simulink model "TST_HLSDem_SelectParameter"  (R2016b)
settings: Solver=FixedStepDiscrete  StartTime=0.0  StopTime=simTime  FixedStep=sampleTime  RelTol=1e-3
values from neighbouring files (symbols this model uses):
  testCase = 1    [initTST_HLSDem_SelectParameter_001.m]    (also in initTST_HLSDem_SelectParameter_002.m = 2; initTST_HLSDem_SelectParameter_003.m = 3; initTST_HLSDem_SelectParameter_004.m = 4; initTST_HLSDem_SelectParameter_005.m = 5)
libraries: simulink x146, UnitTest_Lib x140
(part 1 of 4)
settings Model: Creator=caijinkang  LastModifiedBy=caijinkang
settings DebuggingCC: SignalRangeChecking=error

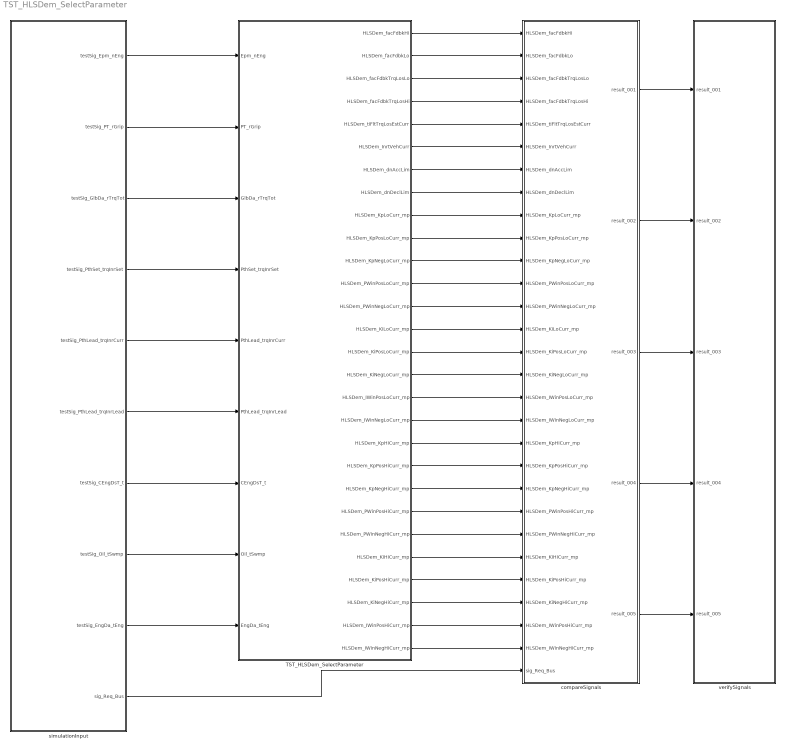
== system TST_HLSDem_SelectParameter ==
  TST_HLSDem_SelectParameter : Subsystem
  compareSignals : Subsystem
  simulationInput : Subsystem
  verifySignals : Subsystem
  wires:
  simulationInput/1(testSig_Epm_nEng) -> TST_HLSDem_SelectParameter/1(Epm_nEng)
  simulationInput/2(testSig_PT_rGrip) -> TST_HLSDem_SelectParameter/2(PT_rGrip)
  simulationInput/3(testSig_GlbDa_rTrqTot) -> TST_HLSDem_SelectParameter/3(GlbDa_rTrqTot)
  simulationInput/4(testSig_PthSet_trqInrSet) -> TST_HLSDem_SelectParameter/4(PthSet_trqInrSet)
  simulationInput/5(testSig_PthLead_trqInrCurr) -> TST_HLSDem_SelectParameter/5(PthLead_trqInrCurr)
  simulationInput/6(testSig_PthLead_trqInrLead) -> TST_HLSDem_SelectParameter/6(PthLead_trqInrLead)
  simulationInput/7(testSig_CEngDsT_t) -> TST_HLSDem_SelectParameter/7(CEngDsT_t)
  simulationInput/8(testSig_Oil_tSwmp) -> TST_HLSDem_SelectParameter/8(Oil_tSwmp)
  simulationInput/9(testSig_EngDa_tEng) -> TST_HLSDem_SelectParameter/9(EngDa_tEng)
  TST_HLSDem_SelectParameter/1(HLSDem_facFdbkHi) -> compareSignals/1(HLSDem_facFdbkHi)
  TST_HLSDem_SelectParameter/2(HLSDem_facFdbkLo) -> compareSignals/2(HLSDem_facFdbkLo)
  TST_HLSDem_SelectParameter/3(HLSDem_facFdbkTrqLosLo) -> compareSignals/3(HLSDem_facFdbkTrqLosLo)
  TST_HLSDem_SelectParameter/4(HLSDem_facFdbkTrqLosHi) -> compareSignals/4(HLSDem_facFdbkTrqLosHi)
  TST_HLSDem_SelectParameter/5(HLSDem_tiFltTrqLosEstCurr) -> compareSignals/5(HLSDem_tiFltTrqLosEstCurr)
  TST_HLSDem_SelectParameter/6(HLSDem_InrtVehCurr) -> compareSignals/6(HLSDem_InrtVehCurr)
  TST_HLSDem_SelectParameter/7(HLSDem_dnAccLim) -> compareSignals/7(HLSDem_dnAccLim)
  TST_HLSDem_SelectParameter/8(HLSDem_dnDeclLim) -> compareSignals/8(HLSDem_dnDeclLim)
  TST_HLSDem_SelectParameter/9(HLSDem_KpLoCurr_mp) -> compareSignals/9(HLSDem_KpLoCurr_mp)
  TST_HLSDem_SelectParameter/10(HLSDem_KpPosLoCurr_mp) -> compareSignals/10(HLSDem_KpPosLoCurr_mp)
  TST_HLSDem_SelectParameter/11(HLSDem_KpNegLoCurr_mp) -> compareSignals/11(HLSDem_KpNegLoCurr_mp)
  TST_HLSDem_SelectParameter/12(HLSDem_PWinPosLoCurr_mp) -> compareSignals/12(HLSDem_PWinPosLoCurr_mp)
  TST_HLSDem_SelectParameter/13(HLSDem_PWinNegLoCurr_mp) -> compareSignals/13(HLSDem_PWinNegLoCurr_mp)
  TST_HLSDem_SelectParameter/14(HLSDem_KiLoCurr_mp) -> compareSignals/14(HLSDem_KiLoCurr_mp)
  TST_HLSDem_SelectParameter/15(HLSDem_KiPosLoCurr_mp) -> compareSignals/15(HLSDem_KiPosLoCurr_mp)
  TST_HLSDem_SelectParameter/16(HLSDem_KiNegLoCurr_mp) -> compareSignals/16(HLSDem_KiNegLoCurr_mp)
  TST_HLSDem_SelectParameter/17(HLSDem_IWinPosLoCurr_mp) -> compareSignals/17(HLSDem_IWinPosLoCurr_mp)
  TST_HLSDem_SelectParameter/18(HLSDem_IWinNegLoCurr_mp) -> compareSignals/18(HLSDem_IWinNegLoCurr_mp)
  TST_HLSDem_SelectParameter/19(HLSDem_KpHiCurr_mp) -> compareSignals/19(HLSDem_KpHiCurr_mp)
  TST_HLSDem_SelectParameter/20(HLSDem_KpPosHiCurr_mp) -> compareSignals/20(HLSDem_KpPosHiCurr_mp)
  TST_HLSDem_SelectParameter/21(HLSDem_KpNegHiCurr_mp) -> compareSignals/21(HLSDem_KpNegHiCurr_mp)
  TST_HLSDem_SelectParameter/22(HLSDem_PWinPosHiCurr_mp) -> compareSignals/22(HLSDem_PWinPosHiCurr_mp)
  TST_HLSDem_SelectParameter/23(HLSDem_PWinNegHiCurr_mp) -> compareSignals/23(HLSDem_PWinNegHiCurr_mp)
  TST_HLSDem_SelectParameter/24(HLSDem_KiHiCurr_mp) -> compareSignals/24(HLSDem_KiHiCurr_mp)
  TST_HLSDem_SelectParameter/25(HLSDem_KiPosHiCurr_mp) -> compareSignals/25(HLSDem_KiPosHiCurr_mp)
  TST_HLSDem_SelectParameter/26(HLSDem_KiNegHiCurr_mp) -> compareSignals/26(HLSDem_KiNegHiCurr_mp)
  TST_HLSDem_SelectParameter/27(HLSDem_IWinPosHiCurr_mp) -> compareSignals/27(HLSDem_IWinPosHiCurr_mp)
  TST_HLSDem_SelectParameter/28(HLSDem_IWinNegHiCurr_mp) -> compareSignals/28(HLSDem_IWinNegHiCurr_mp)
  simulationInput/10(sig_Req_Bus) -> compareSignals/29(sig_Req_Bus)
  compareSignals/1(result_001) -> verifySignals/1(result_001)
  compareSignals/2(result_002) -> verifySignals/2(result_002)
  compareSignals/3(result_003) -> verifySignals/3(result_003)
  compareSignals/4(result_004) -> verifySignals/4(result_004)
  compareSignals/5(result_005) -> verifySignals/5(result_005)

== system TST_HLSDem_SelectParameter/TST_HLSDem_SelectParameter ==
  Epm_nEng : Inport
  PT_rGrip : Inport  Port=2
  GlbDa_rTrqTot : Inport  Port=3
  PthSet_trqInrSet : Inport  Port=4
  PthLead_trqInrCurr : Inport  Port=5
  PthLead_trqInrLead : Inport  Port=6
  CEngDsT_t : Inport  Port=7
  Oil_tSwmp : Inport  Port=8
  EngDa_tEng : Inport  Port=9
  Function_Call : simulink/Ports & Subsystems/Function-Call Generator  sample_time=sampleTime  numberOfIterations=1
  HLSDem_SelectParameter : ModelReference  ModelNameDialog=HLSDem_SelectParameter  SimulationMode=Normal  ModelReferenceVersion=1.85  TriggerPortName=function  TriggerPortTriggerType=function-call  TriggerPortStatesWhenEnabling=held
  HLSDem_facFdbkHi : Outport
  HLSDem_facFdbkLo : Outport  Port=2
  HLSDem_facFdbkTrqLosLo : Outport  Port=3
  HLSDem_facFdbkTrqLosHi : Outport  Port=4
  HLSDem_tiFltTrqLosEstCurr : Outport  Port=5
  HLSDem_InrtVehCurr : Outport  Port=6
  HLSDem_dnAccLim : Outport  Port=7
  HLSDem_dnDeclLim : Outport  Port=8
  HLSDem_KpLoCurr_mp : Outport  Port=9
  HLSDem_KpPosLoCurr_mp : Outport  Port=10
  HLSDem_KpNegLoCurr_mp : Outport  Port=11
  HLSDem_PWinPosLoCurr_mp : Outport  Port=12
  HLSDem_PWinNegLoCurr_mp : Outport  Port=13
  HLSDem_KiLoCurr_mp : Outport  Port=14
  HLSDem_KiPosLoCurr_mp : Outport  Port=15
  HLSDem_KiNegLoCurr_mp : Outport  Port=16
  HLSDem_IWinPosLoCurr_mp : Outport  Port=17
  HLSDem_IWinNegLoCurr_mp : Outport  Port=18
  HLSDem_KpHiCurr_mp : Outport  Port=19
  HLSDem_KpPosHiCurr_mp : Outport  Port=20
  HLSDem_KpNegHiCurr_mp : Outport  Port=21
  HLSDem_PWinPosHiCurr_mp : Outport  Port=22
  HLSDem_PWinNegHiCurr_mp : Outport  Port=23
  HLSDem_KiHiCurr_mp : Outport  Port=24
  HLSDem_KiPosHiCurr_mp : Outport  Port=25
  HLSDem_KiNegHiCurr_mp : Outport  Port=26
  HLSDem_IWinPosHiCurr_mp : Outport  Port=27
  HLSDem_IWinNegHiCurr_mp : Outport  Port=28
  wires:
  Function_Call/1 -> HLSDem_SelectParameter/Trigger
  Epm_nEng/1 -> HLSDem_SelectParameter/1
  PT_rGrip/1 -> HLSDem_SelectParameter/2
  GlbDa_rTrqTot/1 -> HLSDem_SelectParameter/3
  PthSet_trqInrSet/1 -> HLSDem_SelectParameter/4
  PthLead_trqInrCurr/1 -> HLSDem_SelectParameter/5
  PthLead_trqInrLead/1 -> HLSDem_SelectParameter/6
  CEngDsT_t/1 -> HLSDem_SelectParameter/7
  Oil_tSwmp/1 -> HLSDem_SelectParameter/8
  EngDa_tEng/1 -> HLSDem_SelectParameter/9
  HLSDem_SelectParameter/1 -> HLSDem_facFdbkHi/1
  HLSDem_SelectParameter/2 -> HLSDem_facFdbkLo/1
  HLSDem_SelectParameter/3 -> HLSDem_facFdbkTrqLosLo/1
  HLSDem_SelectParameter/4 -> HLSDem_facFdbkTrqLosHi/1
  HLSDem_SelectParameter/5 -> HLSDem_tiFltTrqLosEstCurr/1
  HLSDem_SelectParameter/6 -> HLSDem_InrtVehCurr/1
  HLSDem_SelectParameter/7 -> HLSDem_dnAccLim/1
  HLSDem_SelectParameter/8 -> HLSDem_dnDeclLim/1
  HLSDem_SelectParameter/9 -> HLSDem_KpLoCurr_mp/1
  HLSDem_SelectParameter/10 -> HLSDem_KpPosLoCurr_mp/1
  HLSDem_SelectParameter/11 -> HLSDem_KpNegLoCurr_mp/1
  HLSDem_SelectParameter/12 -> HLSDem_PWinPosLoCurr_mp/1
  HLSDem_SelectParameter/13 -> HLSDem_PWinNegLoCurr_mp/1
  HLSDem_SelectParameter/14 -> HLSDem_KiLoCurr_mp/1
  HLSDem_SelectParameter/15 -> HLSDem_KiPosLoCurr_mp/1
  HLSDem_SelectParameter/16 -> HLSDem_KiNegLoCurr_mp/1
  HLSDem_SelectParameter/17 -> HLSDem_IWinPosLoCurr_mp/1
  HLSDem_SelectParameter/18 -> HLSDem_IWinNegLoCurr_mp/1
  HLSDem_SelectParameter/19 -> HLSDem_KpHiCurr_mp/1
  HLSDem_SelectParameter/20 -> HLSDem_KpPosHiCurr_mp/1
  HLSDem_SelectParameter/21 -> HLSDem_KpNegHiCurr_mp/1
  HLSDem_SelectParameter/22 -> HLSDem_PWinPosHiCurr_mp/1
  HLSDem_SelectParameter/23 -> HLSDem_PWinNegHiCurr_mp/1
  HLSDem_SelectParameter/24 -> HLSDem_KiHiCurr_mp/1
  HLSDem_SelectParameter/25 -> HLSDem_KiPosHiCurr_mp/1
  HLSDem_SelectParameter/26 -> HLSDem_KiNegHiCurr_mp/1
  HLSDem_SelectParameter/27 -> HLSDem_IWinPosHiCurr_mp/1
  HLSDem_SelectParameter/28 -> HLSDem_IWinNegHiCurr_mp/1

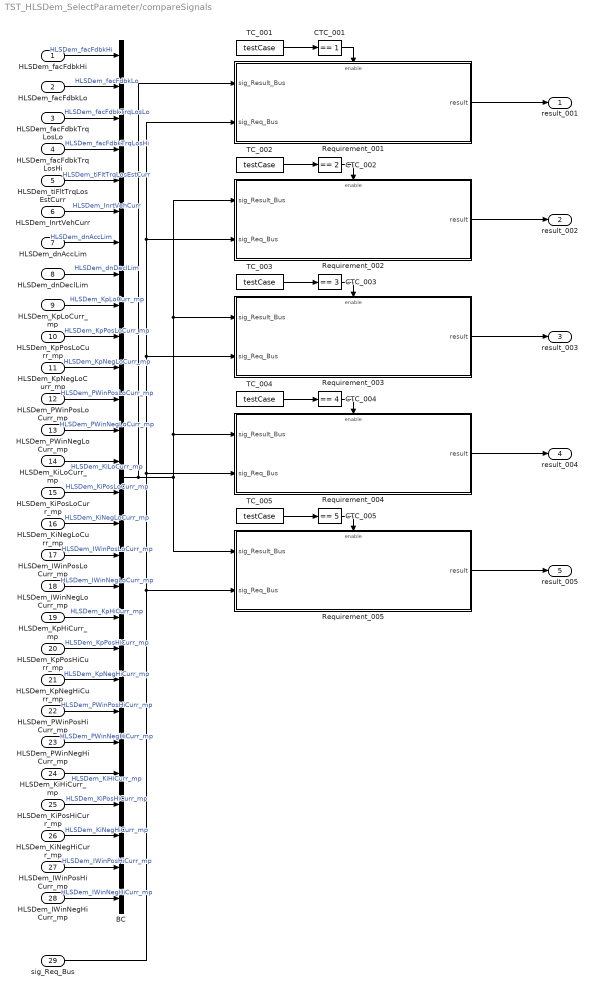
== system TST_HLSDem_SelectParameter/compareSignals ==
  HLSDem_facFdbkHi : Inport
  HLSDem_facFdbkLo : Inport  Port=2
  HLSDem_facFdbkTrqLosLo : Inport  Port=3
  HLSDem_facFdbkTrqLosHi : Inport  Port=4
  HLSDem_tiFltTrqLosEstCurr : Inport  Port=5
  HLSDem_InrtVehCurr : Inport  Port=6
  HLSDem_dnAccLim : Inport  Port=7
  HLSDem_dnDeclLim : Inport  Port=8
  HLSDem_KpLoCurr_mp : Inport  Port=9
  HLSDem_KpPosLoCurr_mp : Inport  Port=10
  HLSDem_KpNegLoCurr_mp : Inport  Port=11
  HLSDem_PWinPosLoCurr_mp : Inport  Port=12
  HLSDem_PWinNegLoCurr_mp : Inport  Port=13
  HLSDem_KiLoCurr_mp : Inport  Port=14
  HLSDem_KiPosLoCurr_mp : Inport  Port=15
  HLSDem_KiNegLoCurr_mp : Inport  Port=16
  HLSDem_IWinPosLoCurr_mp : Inport  Port=17
  HLSDem_IWinNegLoCurr_mp : Inport  Port=18
  HLSDem_KpHiCurr_mp : Inport  Port=19
  HLSDem_KpPosHiCurr_mp : Inport  Port=20
  HLSDem_KpNegHiCurr_mp : Inport  Port=21
  HLSDem_PWinPosHiCurr_mp : Inport  Port=22
  HLSDem_PWinNegHiCurr_mp : Inport  Port=23
  HLSDem_KiHiCurr_mp : Inport  Port=24
  HLSDem_KiPosHiCurr_mp : Inport  Port=25
  HLSDem_KiNegHiCurr_mp : Inport  Port=26
  HLSDem_IWinPosHiCurr_mp : Inport  Port=27
  HLSDem_IWinNegHiCurr_mp : Inport  Port=28
  sig_Req_Bus : Inport  Port=29
  BC : BusCreator  Inputs=28
  CTC_001 : simulink/Logic and Bit Operations/Compare To Constant  relop===  const=1  OutDataTypeStr=boolean
  CTC_002 : simulink/Logic and Bit Operations/Compare To Constant  relop===  const=2  OutDataTypeStr=boolean
  CTC_003 : simulink/Logic and Bit Operations/Compare To Constant  relop===  const=3  OutDataTypeStr=boolean
  CTC_004 : simulink/Logic and Bit Operations/Compare To Constant  relop===  const=4  OutDataTypeStr=boolean
  CTC_005 : simulink/Logic and Bit Operations/Compare To Constant  relop===  const=5  OutDataTypeStr=boolean
  Requirement_001 : Subsystem
  Requirement_002 : Subsystem
  Requirement_003 : Subsystem
  Requirement_004 : Subsystem
  Requirement_005 : Subsystem
  TC_001 : Constant  Value=testCase
  TC_002 : Constant  Value=testCase
  TC_003 : Constant  Value=testCase
  TC_004 : Constant  Value=testCase
  TC_005 : Constant  Value=testCase
  result_001 : Outport
  result_002 : Outport  Port=2
  result_003 : Outport  Port=3
  result_004 : Outport  Port=4
  result_005 : Outport  Port=5
  wires:
  HLSDem_facFdbkHi/1 -> BC/1  "HLSDem_facFdbkHi"
  HLSDem_facFdbkLo/1 -> BC/2  "HLSDem_facFdbkLo"
  HLSDem_facFdbkTrqLosLo/1 -> BC/3  "HLSDem_facFdbkTrqLosLo"
  HLSDem_facFdbkTrqLosHi/1 -> BC/4  "HLSDem_facFdbkTrqLosHi"
  HLSDem_tiFltTrqLosEstCurr/1 -> BC/5  "HLSDem_tiFltTrqLosEstCurr"
  HLSDem_InrtVehCurr/1 -> BC/6  "HLSDem_InrtVehCurr"
  HLSDem_dnAccLim/1 -> BC/7  "HLSDem_dnAccLim"
  HLSDem_dnDeclLim/1 -> BC/8  "HLSDem_dnDeclLim"
  HLSDem_KpLoCurr_mp/1 -> BC/9  "HLSDem_KpLoCurr_mp"
  HLSDem_KpPosLoCurr_mp/1 -> BC/10  "HLSDem_KpPosLoCurr_mp"
  HLSDem_KpNegLoCurr_mp/1 -> BC/11  "HLSDem_KpNegLoCurr_mp"
  HLSDem_PWinPosLoCurr_mp/1 -> BC/12  "HLSDem_PWinPosLoCurr_mp"
  HLSDem_PWinNegLoCurr_mp/1 -> BC/13  "HLSDem_PWinNegLoCurr_mp"
  HLSDem_KiLoCurr_mp/1 -> BC/14  "HLSDem_KiLoCurr_mp"
  HLSDem_KiPosLoCurr_mp/1 -> BC/15  "HLSDem_KiPosLoCurr_mp"
  HLSDem_KiNegLoCurr_mp/1 -> BC/16  "HLSDem_KiNegLoCurr_mp"
  HLSDem_IWinPosLoCurr_mp/1 -> BC/17  "HLSDem_IWinPosLoCurr_mp"
  HLSDem_IWinNegLoCurr_mp/1 -> BC/18  "HLSDem_IWinNegLoCurr_mp"
  HLSDem_KpHiCurr_mp/1 -> BC/19  "HLSDem_KpHiCurr_mp"
  HLSDem_KpPosHiCurr_mp/1 -> BC/20  "HLSDem_KpPosHiCurr_mp"
  HLSDem_KpNegHiCurr_mp/1 -> BC/21  "HLSDem_KpNegHiCurr_mp"
  HLSDem_PWinPosHiCurr_mp/1 -> BC/22  "HLSDem_PWinPosHiCurr_mp"
  HLSDem_PWinNegHiCurr_mp/1 -> BC/23  "HLSDem_PWinNegHiCurr_mp"
  HLSDem_KiHiCurr_mp/1 -> BC/24  "HLSDem_KiHiCurr_mp"
  HLSDem_KiPosHiCurr_mp/1 -> BC/25  "HLSDem_KiPosHiCurr_mp"
  HLSDem_KiNegHiCurr_mp/1 -> BC/26  "HLSDem_KiNegHiCurr_mp"
  HLSDem_IWinPosHiCurr_mp/1 -> BC/27  "HLSDem_IWinPosHiCurr_mp"
  HLSDem_IWinNegHiCurr_mp/1 -> BC/28  "HLSDem_IWinNegHiCurr_mp"
  TC_001/1 -> CTC_001/1
  CTC_001/1 -> Requirement_001/Enable
  sig_Req_Bus/1 -> Requirement_001/2(sig_Req_Bus), Requirement_002/2(sig_Req_Bus), Requirement_003/2(sig_Req_Bus), Requirement_004/2(sig_Req_Bus), Requirement_005/2(sig_Req_Bus)
  BC/1 -> Requirement_002/1(sig_Result_Bus), Requirement_003/1(sig_Result_Bus), Requirement_004/1(sig_Result_Bus), Requirement_005/1(sig_Result_Bus), Requirement_001/1(sig_Result_Bus)
  Requirement_001/1(result) -> result_001/1
  TC_002/1 -> CTC_002/1
  CTC_002/1 -> Requirement_002/Enable
  Requirement_002/1(result) -> result_002/1
  TC_003/1 -> CTC_003/1
  CTC_003/1 -> Requirement_003/Enable
  Requirement_003/1(result) -> result_003/1
  TC_004/1 -> CTC_004/1
  CTC_004/1 -> Requirement_004/Enable
  Requirement_004/1(result) -> result_004/1
  TC_005/1 -> CTC_005/1
  CTC_005/1 -> Requirement_005/Enable
  Requirement_005/1(result) -> result_005/1

== system TST_HLSDem_SelectParameter/simulationInput ==
  BS : BusSelector  OutputSignals=testSig_Epm_nEng,testSig_PT_rGrip,testSig_GlbDa_rTrqTot,testSig_PthSet_trqInrSet,testSig_PthLead_trqInrCurr,testSig_PthLead_trqInrLead,testSig_CEngDsT_t,testSig_Oil_tSwmp,testSig_EngDa_tEng
  MPSw : MultiPortSwitch  Inputs=5  SaturateOnIntegerOverflow=on  InputSameDT=on
  TestCase : Constant  Value=testCase
  testSignals_R001 : Subsystem
  testSignals_R002 : Subsystem
  testSignals_R003 : Subsystem
  testSignals_R004 : Subsystem
  testSignals_R005 : Subsystem
  testSig_Epm_nEng : Outport
  testSig_PT_rGrip : Outport  Port=2
  testSig_GlbDa_rTrqTot : Outport  Port=3
  testSig_PthSet_trqInrSet : Outport  Port=4
  testSig_PthLead_trqInrCurr : Outport  Port=5
  testSig_PthLead_trqInrLead : Outport  Port=6
  testSig_CEngDsT_t : Outport  Port=7
  testSig_Oil_tSwmp : Outport  Port=8
  testSig_EngDa_tEng : Outport  Port=9
  sig_Req_Bus : Outport  Port=10
  wires:
  BS/1 -> testSig_Epm_nEng/1  "<testSig_Epm_nEng>"
  BS/2 -> testSig_PT_rGrip/1  "<testSig_PT_rGrip>"
  BS/3 -> testSig_GlbDa_rTrqTot/1  "<testSig_GlbDa_rTrqTot>"
  BS/4 -> testSig_PthSet_trqInrSet/1  "<testSig_PthSet_trqInrSet>"
  BS/5 -> testSig_PthLead_trqInrCurr/1  "<testSig_PthLead_trqInrCurr>"
  BS/6 -> testSig_PthLead_trqInrLead/1  "<testSig_PthLead_trqInrLead>"
  BS/7 -> testSig_CEngDsT_t/1  "<testSig_CEngDsT_t>"
  BS/8 -> testSig_Oil_tSwmp/1  "<testSig_Oil_tSwmp>"
  BS/9 -> testSig_EngDa_tEng/1  "<testSig_EngDa_tEng>"
  MPSw/1 -> BS/1, sig_Req_Bus/1
  TestCase/1 -> MPSw/1
  testSignals_R001/1(testSignals) -> MPSw/2
  testSignals_R002/1(testSignals) -> MPSw/3
  testSignals_R003/1(testSignals) -> MPSw/4
  testSignals_R004/1(testSignals) -> MPSw/5
  testSignals_R005/1(testSignals) -> MPSw/6

== system TST_HLSDem_SelectParameter/verifySignals ==
  result_001 : Inport
  result_002 : Inport  Port=2
  result_003 : Inport  Port=3
  result_004 : Inport  Port=4
  result_005 : Inport  Port=5
  Assertion_001 : Assertion  Enabled=off
  Assertion_002 : Assertion  Enabled=off
  Assertion_003 : Assertion  Enabled=off
  Assertion_004 : Assertion  Enabled=off
  Assertion_005 : Assertion  Enabled=off
  wires:
  result_001/1 -> Assertion_001/1
  result_002/1 -> Assertion_002/1
  result_003/1 -> Assertion_003/1
  result_004/1 -> Assertion_004/1
  result_005/1 -> Assertion_005/1

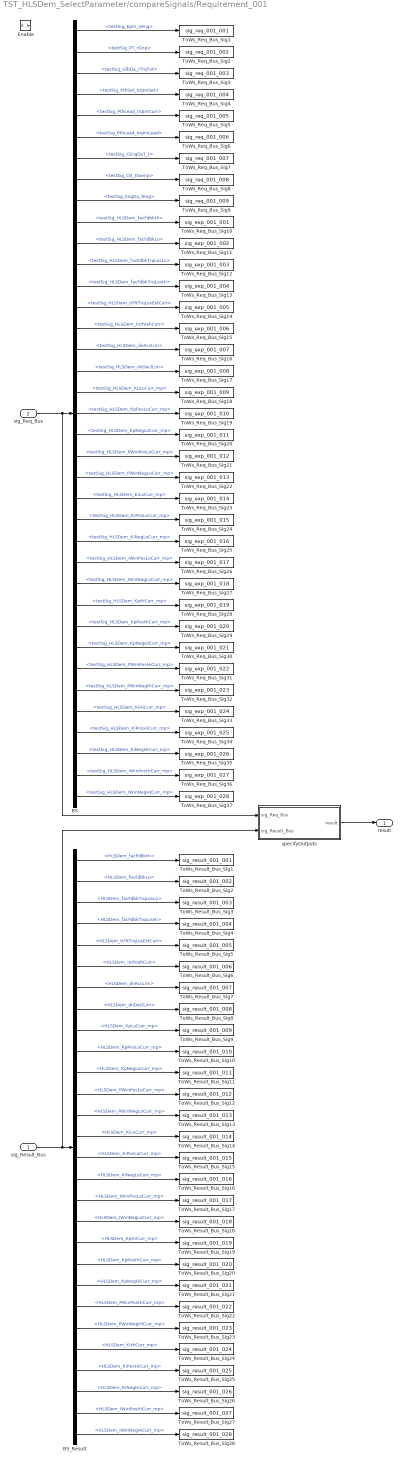
== system TST_HLSDem_SelectParameter/compareSignals/Requirement_001 ==
  sig_Result_Bus : Inport
  sig_Req_Bus : Inport  Port=2
  Enable : EnablePort
  BS : BusSelector  OutputSignals=testSig_Epm_nEng,testSig_PT_rGrip,testSig_GlbDa_rTrqTot,testSig_PthSet_trqInrSet,testSig_PthLead_trqInrCurr,testSig_PthLead_trqInrLead,testSig_CEngDsT_t,testSig_Oil_tSwmp,testSig_EngDa_tEng,testSig_HLSDem_facFdbkHi,testSig_HLSDem_facFdbkLo,testSig_HLSDem_facFdbkTrqLosLo,testSig_HLSDem_facFdbkTrqLosHi,testSig_HLSDem_tiFltTrqLosEstCurr,testSig_HLSDem_InrtVehCurr,testSig_HLSDem_dnAccLim,testSig_HLSDem_dnDeclLim,testSig_HLSDem_KpLoCurr_mp,testSig_HLSDem_KpPosLoCurr_mp,testSig_HLSDem_KpNegLoCurr_mp,testSig_HLSDem_PWinPosLoCurr_mp,testSig_HLSDem_PWinNegLoCurr_mp,testSig_HLSDem_KiLoCurr_mp,testSig_HLSDem_KiPosLoCurr_mp,testSig_HLSDem_KiNegLoCurr_mp,testSig_HLSDem_IWinPosLoCurr_mp,testSig_HLSDem_IWinNegLoCurr_mp,testSig_HLSDem_KpHiCurr_mp,testSig_HLSDem_KpPosHiCurr_mp,testSig_HLSDem_KpNegHiCurr_mp,testSig_HLSDem_PWinPosHiCurr_mp,testSig_HLSDem_PWinNegHiCurr_mp,testSig_HLSDem_KiHiCurr_mp,testSig_HLSDem_KiPosHiCurr_mp,testSig_HLSDem_KiNegHiCurr_mp,testSig_HLSDem_IWinPosHiCurr_mp,testSig_HLSDem_IWinNegHiCurr_mp
  BS_Result : BusSelector  OutputSignals=HLSDem_facFdbkHi,HLSDem_facFdbkLo,HLSDem_facFdbkTrqLosLo,HLSDem_facFdbkTrqLosHi,HLSDem_tiFltTrqLosEstCurr,HLSDem_InrtVehCurr,HLSDem_dnAccLim,HLSDem_dnDeclLim,HLSDem_KpLoCurr_mp,HLSDem_KpPosLoCurr_mp,HLSDem_KpNegLoCurr_mp,HLSDem_PWinPosLoCurr_mp,HLSDem_PWinNegLoCurr_mp,HLSDem_KiLoCurr_mp,HLSDem_KiPosLoCurr_mp,HLSDem_KiNegLoCurr_mp,HLSDem_IWinPosLoCurr_mp,HLSDem_IWinNegLoCurr_mp,HLSDem_KpHiCurr_mp,HLSDem_KpPosHiCurr_mp,HLSDem_KpNegHiCurr_mp,HLSDem_PWinPosHiCurr_mp,HLSDem_PWinNegHiCurr_mp,HLSDem_KiHiCurr_mp,HLSDem_KiPosHiCurr_mp,HLSDem_KiNegHiCurr_mp,HLSDem_IWinPosHiCurr_mp,HLSDem_IWinNegHiCurr_mp
  ToWs_Req_Bus_Sig1 : ToWorkspace  VariableName=sig_req_001_001  SaveFormat=Structure With Time
  ToWs_Req_Bus_Sig10 : ToWorkspace  VariableName=sig_exp_001_001  SaveFormat=Structure With Time
  ToWs_Req_Bus_Sig11 : ToWorkspace  VariableName=sig_exp_001_002  SaveFormat=Structure With Time
  ToWs_Req_Bus_Sig12 : ToWorkspace  VariableName=sig_exp_001_003  SaveFormat=Structure With Time
  ToWs_Req_Bus_Sig13 : ToWorkspace  VariableName=sig_exp_001_004  SaveFormat=Structure With Time
  ToWs_Req_Bus_Sig14 : ToWorkspace  VariableName=sig_exp_001_005  SaveFormat=Structure With Time
  ToWs_Req_Bus_Sig15 : ToWorkspace  VariableName=sig_exp_001_006  SaveFormat=Structure With Time
  ToWs_Req_Bus_Sig16 : ToWorkspace  VariableName=sig_exp_001_007  SaveFormat=Structure With Time
  ToWs_Req_Bus_Sig17 : ToWorkspace  VariableName=sig_exp_001_008  SaveFormat=Structure With Time
  ToWs_Req_Bus_Sig18 : ToWorkspace  VariableName=sig_exp_001_009  SaveFormat=Structure With Time
  ToWs_Req_Bus_Sig19 : ToWorkspace  VariableName=sig_exp_001_010  SaveFormat=Structure With Time
  ToWs_Req_Bus_Sig2 : ToWorkspace  VariableName=sig_req_001_002  SaveFormat=Structure With Time
  ToWs_Req_Bus_Sig20 : ToWorkspace  VariableName=sig_exp_001_011  SaveFormat=Structure With Time
  ToWs_Req_Bus_Sig21 : ToWorkspace  VariableName=sig_exp_001_012  SaveFormat=Structure With Time
  ToWs_Req_Bus_Sig22 : ToWorkspace  VariableName=sig_exp_001_013  SaveFormat=Structure With Time
  ToWs_Req_Bus_Sig23 : ToWorkspace  VariableName=sig_exp_001_014  SaveFormat=Structure With Time
  ToWs_Req_Bus_Sig24 : ToWorkspace  VariableName=sig_exp_001_015  SaveFormat=Structure With Time
  ToWs_Req_Bus_Sig25 : ToWorkspace  VariableName=sig_exp_001_016  SaveFormat=Structure With Time
  ToWs_Req_Bus_Sig26 : ToWorkspace  VariableName=sig_exp_001_017  SaveFormat=Structure With Time
  ToWs_Req_Bus_Sig27 : ToWorkspace  VariableName=sig_exp_001_018  SaveFormat=Structure With Time
  ToWs_Req_Bus_Sig28 : ToWorkspace  VariableName=sig_exp_001_019  SaveFormat=Structure With Time
  ToWs_Req_Bus_Sig29 : ToWorkspace  VariableName=sig_exp_001_020  SaveFormat=Structure With Time
  ToWs_Req_Bus_Sig3 : ToWorkspace  VariableName=sig_req_001_003  SaveFormat=Structure With Time
  ToWs_Req_Bus_Sig30 : ToWorkspace  VariableName=sig_exp_001_021  SaveFormat=Structure With Time
  ToWs_Req_Bus_Sig31 : ToWorkspace  VariableName=sig_exp_001_022  SaveFormat=Structure With Time
  ToWs_Req_Bus_Sig32 : ToWorkspace  VariableName=sig_exp_001_023  SaveFormat=Structure With Time
  ToWs_Req_Bus_Sig33 : ToWorkspace  VariableName=sig_exp_001_024  SaveFormat=Structure With Time
  ToWs_Req_Bus_Sig34 : ToWorkspace  VariableName=sig_exp_001_025  SaveFormat=Structure With Time
  ToWs_Req_Bus_Sig35 : ToWorkspace  VariableName=sig_exp_001_026  SaveFormat=Structure With Time
  ToWs_Req_Bus_Sig36 : ToWorkspace  VariableName=sig_exp_001_027  SaveFormat=Structure With Time
  ToWs_Req_Bus_Sig37 : ToWorkspace  VariableName=sig_exp_001_028  SaveFormat=Structure With Time
  ToWs_Req_Bus_Sig4 : ToWorkspace  VariableName=sig_req_001_004  SaveFormat=Structure With Time
  ToWs_Req_Bus_Sig5 : ToWorkspace  VariableName=sig_req_001_005  SaveFormat=Structure With Time
  ToWs_Req_Bus_Sig6 : ToWorkspace  VariableName=sig_req_001_006  SaveFormat=Structure With Time
  ToWs_Req_Bus_Sig7 : ToWorkspace  VariableName=sig_req_001_007  SaveFormat=Structure With Time
  ToWs_Req_Bus_Sig8 : ToWorkspace  VariableName=sig_req_001_008  SaveFormat=Structure With Time
  ToWs_Req_Bus_Sig9 : ToWorkspace  VariableName=sig_req_001_009  SaveFormat=Structure With Time
  ToWs_Result_Bus_Sig1 : ToWorkspace  VariableName=sig_result_001_001  SaveFormat=Structure With Time
  ToWs_Result_Bus_Sig10 : ToWorkspace  VariableName=sig_result_001_010  SaveFormat=Structure With Time
  ToWs_Result_Bus_Sig11 : ToWorkspace  VariableName=sig_result_001_011  SaveFormat=Structure With Time
  ToWs_Result_Bus_Sig12 : ToWorkspace  VariableName=sig_result_001_012  SaveFormat=Structure With Time
  ToWs_Result_Bus_Sig13 : ToWorkspace  VariableName=sig_result_001_013  SaveFormat=Structure With Time
  ToWs_Result_Bus_Sig14 : ToWorkspace  VariableName=sig_result_001_014  SaveFormat=Structure With Time
  ToWs_Result_Bus_Sig15 : ToWorkspace  VariableName=sig_result_001_015  SaveFormat=Structure With Time
  ToWs_Result_Bus_Sig16 : ToWorkspace  VariableName=sig_result_001_016  SaveFormat=Structure With Time
  ToWs_Result_Bus_Sig17 : ToWorkspace  VariableName=sig_result_001_017  SaveFormat=Structure With Time
  ToWs_Result_Bus_Sig18 : ToWorkspace  VariableName=sig_result_001_018  SaveFormat=Structure With Time
  ToWs_Result_Bus_Sig19 : ToWorkspace  VariableName=sig_result_001_019  SaveFormat=Structure With Time
  ToWs_Result_Bus_Sig2 : ToWorkspace  VariableName=sig_result_001_002  SaveFormat=Structure With Time
  ToWs_Result_Bus_Sig20 : ToWorkspace  VariableName=sig_result_001_020  SaveFormat=Structure With Time
  ToWs_Result_Bus_Sig21 : ToWorkspace  VariableName=sig_result_001_021  SaveFormat=Structure With Time
  ToWs_Result_Bus_Sig22 : ToWorkspace  VariableName=sig_result_001_022  SaveFormat=Structure With Time
  ToWs_Result_Bus_Sig23 : ToWorkspace  VariableName=sig_result_001_023  SaveFormat=Structure With Time
  ToWs_Result_Bus_Sig24 : ToWorkspace  VariableName=sig_result_001_024  SaveFormat=Structure With Time
  ToWs_Result_Bus_Sig25 : ToWorkspace  VariableName=sig_result_001_025  SaveFormat=Structure With Time
  ToWs_Result_Bus_Sig26 : ToWorkspace  VariableName=sig_result_001_026  SaveFormat=Structure With Time
  ToWs_Result_Bus_Sig27 : ToWorkspace  VariableName=sig_result_001_027  SaveFormat=Structure With Time
  ToWs_Result_Bus_Sig28 : ToWorkspace  VariableName=sig_result_001_028  SaveFormat=Structure With Time
  ToWs_Result_Bus_Sig3 : ToWorkspace  VariableName=sig_result_001_003  SaveFormat=Structure With Time
  ToWs_Result_Bus_Sig4 : ToWorkspace  VariableName=sig_result_001_004  SaveFormat=Structure With Time
  ToWs_Result_Bus_Sig5 : ToWorkspace  VariableName=sig_result_001_005  SaveFormat=Structure With Time
  ToWs_Result_Bus_Sig6 : ToWorkspace  VariableName=sig_result_001_006  SaveFormat=Structure With Time
  ToWs_Result_Bus_Sig7 : ToWorkspace  VariableName=sig_result_001_007  SaveFormat=Structure With Time
  ToWs_Result_Bus_Sig8 : ToWorkspace  VariableName=sig_result_001_008  SaveFormat=Structure With Time
  ToWs_Result_Bus_Sig9 : ToWorkspace  VariableName=sig_result_001_009  SaveFormat=Structure With Time
  specifyOutputs : Subsystem
  result : Outport
  wires:
  sig_Req_Bus/1 -> BS/1, specifyOutputs/1(sig_Req_Bus)
  BS/1 -> ToWs_Req_Bus_Sig1/1  "<testSig_Epm_nEng>"
  BS/2 -> ToWs_Req_Bus_Sig2/1  "<testSig_PT_rGrip>"
  BS/3 -> ToWs_Req_Bus_Sig3/1  "<testSig_GlbDa_rTrqTot>"
  BS/4 -> ToWs_Req_Bus_Sig4/1  "<testSig_PthSet_trqInrSet>"
  BS/5 -> ToWs_Req_Bus_Sig5/1  "<testSig_PthLead_trqInrCurr>"
  BS/6 -> ToWs_Req_Bus_Sig6/1  "<testSig_PthLead_trqInrLead>"
  BS/7 -> ToWs_Req_Bus_Sig7/1  "<testSig_CEngDsT_t>"
  BS/8 -> ToWs_Req_Bus_Sig8/1  "<testSig_Oil_tSwmp>"
  BS/9 -> ToWs_Req_Bus_Sig9/1  "<testSig_EngDa_tEng>"
  BS/10 -> ToWs_Req_Bus_Sig10/1  "<testSig_HLSDem_facFdbkHi>"
  BS/11 -> ToWs_Req_Bus_Sig11/1  "<testSig_HLSDem_facFdbkLo>"
  BS/12 -> ToWs_Req_Bus_Sig12/1  "<testSig_HLSDem_facFdbkTrqLosLo>"
  BS/13 -> ToWs_Req_Bus_Sig13/1  "<testSig_HLSDem_facFdbkTrqLosHi>"
  BS/14 -> ToWs_Req_Bus_Sig14/1  "<testSig_HLSDem_tiFltTrqLosEstCurr>"
  BS/15 -> ToWs_Req_Bus_Sig15/1  "<testSig_HLSDem_InrtVehCurr>"
  BS/16 -> ToWs_Req_Bus_Sig16/1  "<testSig_HLSDem_dnAccLim>"
  BS/17 -> ToWs_Req_Bus_Sig17/1  "<testSig_HLSDem_dnDeclLim>"
  BS/18 -> ToWs_Req_Bus_Sig18/1  "<testSig_HLSDem_KpLoCurr_mp>"
  BS/19 -> ToWs_Req_Bus_Sig19/1  "<testSig_HLSDem_KpPosLoCurr_mp>"
  BS/20 -> ToWs_Req_Bus_Sig20/1  "<testSig_HLSDem_KpNegLoCurr_mp>"
  BS/21 -> ToWs_Req_Bus_Sig21/1  "<testSig_HLSDem_PWinPosLoCurr_mp>"
  BS/22 -> ToWs_Req_Bus_Sig22/1  "<testSig_HLSDem_PWinNegLoCurr_mp>"
  BS/23 -> ToWs_Req_Bus_Sig23/1  "<testSig_HLSDem_KiLoCurr_mp>"
  BS/24 -> ToWs_Req_Bus_Sig24/1  "<testSig_HLSDem_KiPosLoCurr_mp>"
  BS/25 -> ToWs_Req_Bus_Sig25/1  "<testSig_HLSDem_KiNegLoCurr_mp>"
  BS/26 -> ToWs_Req_Bus_Sig26/1  "<testSig_HLSDem_IWinPosLoCurr_mp>"
  BS/27 -> ToWs_Req_Bus_Sig27/1  "<testSig_HLSDem_IWinNegLoCurr_mp>"
  BS/28 -> ToWs_Req_Bus_Sig28/1  "<testSig_HLSDem_KpHiCurr_mp>"
  BS/29 -> ToWs_Req_Bus_Sig29/1  "<testSig_HLSDem_KpPosHiCurr_mp>"
  BS/30 -> ToWs_Req_Bus_Sig30/1  "<testSig_HLSDem_KpNegHiCurr_mp>"
  BS/31 -> ToWs_Req_Bus_Sig31/1  "<testSig_HLSDem_PWinPosHiCurr_mp>"
  BS/32 -> ToWs_Req_Bus_Sig32/1  "<testSig_HLSDem_PWinNegHiCurr_mp>"
  BS/33 -> ToWs_Req_Bus_Sig33/1  "<testSig_HLSDem_KiHiCurr_mp>"
  BS/34 -> ToWs_Req_Bus_Sig34/1  "<testSig_HLSDem_KiPosHiCurr_mp>"
  BS/35 -> ToWs_Req_Bus_Sig35/1  "<testSig_HLSDem_KiNegHiCurr_mp>"
  BS/36 -> ToWs_Req_Bus_Sig36/1  "<testSig_HLSDem_IWinPosHiCurr_mp>"
  BS/37 -> ToWs_Req_Bus_Sig37/1  "<testSig_HLSDem_IWinNegHiCurr_mp>"
  sig_Result_Bus/1 -> BS_Result/1, specifyOutputs/2(sig_Result_Bus)
  BS_Result/1 -> ToWs_Result_Bus_Sig1/1  "<HLSDem_facFdbkHi>"
  BS_Result/2 -> ToWs_Result_Bus_Sig2/1  "<HLSDem_facFdbkLo>"
  BS_Result/3 -> ToWs_Result_Bus_Sig3/1  "<HLSDem_facFdbkTrqLosLo>"
  BS_Result/4 -> ToWs_Result_Bus_Sig4/1  "<HLSDem_facFdbkTrqLosHi>"
  BS_Result/5 -> ToWs_Result_Bus_Sig5/1  "<HLSDem_tiFltTrqLosEstCurr>"
  BS_Result/6 -> ToWs_Result_Bus_Sig6/1  "<HLSDem_InrtVehCurr>"
  BS_Result/7 -> ToWs_Result_Bus_Sig7/1  "<HLSDem_dnAccLim>"
  BS_Result/8 -> ToWs_Result_Bus_Sig8/1  "<HLSDem_dnDeclLim>"
  BS_Result/9 -> ToWs_Result_Bus_Sig9/1  "<HLSDem_KpLoCurr_mp>"
  BS_Result/10 -> ToWs_Result_Bus_Sig10/1  "<HLSDem_KpPosLoCurr_mp>"
  BS_Result/11 -> ToWs_Result_Bus_Sig11/1  "<HLSDem_KpNegLoCurr_mp>"
  BS_Result/12 -> ToWs_Result_Bus_Sig12/1  "<HLSDem_PWinPosLoCurr_mp>"
  BS_Result/13 -> ToWs_Result_Bus_Sig13/1  "<HLSDem_PWinNegLoCurr_mp>"
  BS_Result/14 -> ToWs_Result_Bus_Sig14/1  "<HLSDem_KiLoCurr_mp>"
  BS_Result/15 -> ToWs_Result_Bus_Sig15/1  "<HLSDem_KiPosLoCurr_mp>"
  BS_Result/16 -> ToWs_Result_Bus_Sig16/1  "<HLSDem_KiNegLoCurr_mp>"
  BS_Result/17 -> ToWs_Result_Bus_Sig17/1  "<HLSDem_IWinPosLoCurr_mp>"
  BS_Result/18 -> ToWs_Result_Bus_Sig18/1  "<HLSDem_IWinNegLoCurr_mp>"
  BS_Result/19 -> ToWs_Result_Bus_Sig19/1  "<HLSDem_KpHiCurr_mp>"
  BS_Result/20 -> ToWs_Result_Bus_Sig20/1  "<HLSDem_KpPosHiCurr_mp>"
  BS_Result/21 -> ToWs_Result_Bus_Sig21/1  "<HLSDem_KpNegHiCurr_mp>"
  BS_Result/22 -> ToWs_Result_Bus_Sig22/1  "<HLSDem_PWinPosHiCurr_mp>"
  BS_Result/23 -> ToWs_Result_Bus_Sig23/1  "<HLSDem_PWinNegHiCurr_mp>"
  BS_Result/24 -> ToWs_Result_Bus_Sig24/1  "<HLSDem_KiHiCurr_mp>"
  BS_Result/25 -> ToWs_Result_Bus_Sig25/1  "<HLSDem_KiPosHiCurr_mp>"
  BS_Result/26 -> ToWs_Result_Bus_Sig26/1  "<HLSDem_KiNegHiCurr_mp>"
  BS_Result/27 -> ToWs_Result_Bus_Sig27/1  "<HLSDem_IWinPosHiCurr_mp>"
  BS_Result/28 -> ToWs_Result_Bus_Sig28/1  "<HLSDem_IWinNegHiCurr_mp>"
  specifyOutputs/1(result) -> result/1

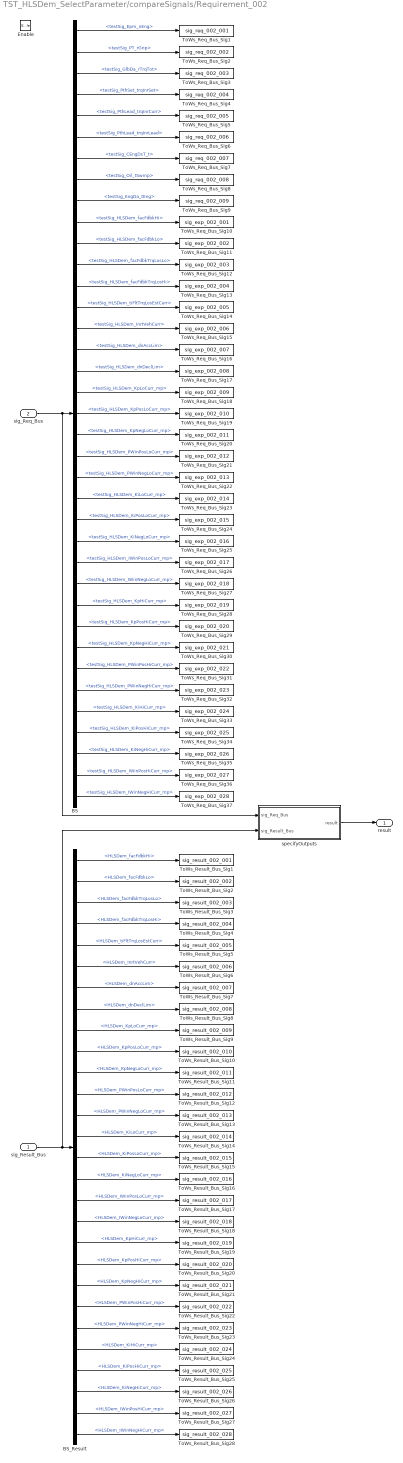
== system TST_HLSDem_SelectParameter/compareSignals/Requirement_002 ==
  sig_Result_Bus : Inport
  sig_Req_Bus : Inport  Port=2
  Enable : EnablePort
  BS : BusSelector  OutputSignals=testSig_Epm_nEng,testSig_PT_rGrip,testSig_GlbDa_rTrqTot,testSig_PthSet_trqInrSet,testSig_PthLead_trqInrCurr,testSig_PthLead_trqInrLead,testSig_CEngDsT_t,testSig_Oil_tSwmp,testSig_EngDa_tEng,testSig_HLSDem_facFdbkHi,testSig_HLSDem_facFdbkLo,testSig_HLSDem_facFdbkTrqLosLo,testSig_HLSDem_facFdbkTrqLosHi,testSig_HLSDem_tiFltTrqLosEstCurr,testSig_HLSDem_InrtVehCurr,testSig_HLSDem_dnAccLim,testSig_HLSDem_dnDeclLim,testSig_HLSDem_KpLoCurr_mp,testSig_HLSDem_KpPosLoCurr_mp,testSig_HLSDem_KpNegLoCurr_mp,testSig_HLSDem_PWinPosLoCurr_mp,testSig_HLSDem_PWinNegLoCurr_mp,testSig_HLSDem_KiLoCurr_mp,testSig_HLSDem_KiPosLoCurr_mp,testSig_HLSDem_KiNegLoCurr_mp,testSig_HLSDem_IWinPosLoCurr_mp,testSig_HLSDem_IWinNegLoCurr_mp,testSig_HLSDem_KpHiCurr_mp,testSig_HLSDem_KpPosHiCurr_mp,testSig_HLSDem_KpNegHiCurr_mp,testSig_HLSDem_PWinPosHiCurr_mp,testSig_HLSDem_PWinNegHiCurr_mp,testSig_HLSDem_KiHiCurr_mp,testSig_HLSDem_KiPosHiCurr_mp,testSig_HLSDem_KiNegHiCurr_mp,testSig_HLSDem_IWinPosHiCurr_mp,testSig_HLSDem_IWinNegHiCurr_mp
  BS_Result : BusSelector  OutputSignals=HLSDem_facFdbkHi,HLSDem_facFdbkLo,HLSDem_facFdbkTrqLosLo,HLSDem_facFdbkTrqLosHi,HLSDem_tiFltTrqLosEstCurr,HLSDem_InrtVehCurr,HLSDem_dnAccLim,HLSDem_dnDeclLim,HLSDem_KpLoCurr_mp,HLSDem_KpPosLoCurr_mp,HLSDem_KpNegLoCurr_mp,HLSDem_PWinPosLoCurr_mp,HLSDem_PWinNegLoCurr_mp,HLSDem_KiLoCurr_mp,HLSDem_KiPosLoCurr_mp,HLSDem_KiNegLoCurr_mp,HLSDem_IWinPosLoCurr_mp,HLSDem_IWinNegLoCurr_mp,HLSDem_KpHiCurr_mp,HLSDem_KpPosHiCurr_mp,HLSDem_KpNegHiCurr_mp,HLSDem_PWinPosHiCurr_mp,HLSDem_PWinNegHiCurr_mp,HLSDem_KiHiCurr_mp,HLSDem_KiPosHiCurr_mp,HLSDem_KiNegHiCurr_mp,HLSDem_IWinPosHiCurr_mp,HLSDem_IWinNegHiCurr_mp
  ToWs_Req_Bus_Sig1 : ToWorkspace  VariableName=sig_req_002_001  SaveFormat=Structure With Time
  ToWs_Req_Bus_Sig10 : ToWorkspace  VariableName=sig_exp_002_001  SaveFormat=Structure With Time
  ToWs_Req_Bus_Sig11 : ToWorkspace  VariableName=sig_exp_002_002  SaveFormat=Structure With Time
  ToWs_Req_Bus_Sig12 : ToWorkspace  VariableName=sig_exp_002_003  SaveFormat=Structure With Time
  ToWs_Req_Bus_Sig13 : ToWorkspace  VariableName=sig_exp_002_004  SaveFormat=Structure With Time
  ToWs_Req_Bus_Sig14 : ToWorkspace  VariableName=sig_exp_002_005  SaveFormat=Structure With Time
  ToWs_Req_Bus_Sig15 : ToWorkspace  VariableName=sig_exp_002_006  SaveFormat=Structure With Time
  ToWs_Req_Bus_Sig16 : ToWorkspace  VariableName=sig_exp_002_007  SaveFormat=Structure With Time
  ToWs_Req_Bus_Sig17 : ToWorkspace  VariableName=sig_exp_002_008  SaveFormat=Structure With Time
  ToWs_Req_Bus_Sig18 : ToWorkspace  VariableName=sig_exp_002_009  SaveFormat=Structure With Time
  ToWs_Req_Bus_Sig19 : ToWorkspace  VariableName=sig_exp_002_010  SaveFormat=Structure With Time
  ToWs_Req_Bus_Sig2 : ToWorkspace  VariableName=sig_req_002_002  SaveFormat=Structure With Time
  ToWs_Req_Bus_Sig20 : ToWorkspace  VariableName=sig_exp_002_011  SaveFormat=Structure With Time
  ToWs_Req_Bus_Sig21 : ToWorkspace  VariableName=sig_exp_002_012  SaveFormat=Structure With Time
  ToWs_Req_Bus_Sig22 : ToWorkspace  VariableName=sig_exp_002_013  SaveFormat=Structure With Time
  ToWs_Req_Bus_Sig23 : ToWorkspace  VariableName=sig_exp_002_014  SaveFormat=Structure With Time
  ToWs_Req_Bus_Sig24 : ToWorkspace  VariableName=sig_exp_002_015  SaveFormat=Structure With Time
  ToWs_Req_Bus_Sig25 : ToWorkspace  VariableName=sig_exp_002_016  SaveFormat=Structure With Time
  ToWs_Req_Bus_Sig26 : ToWorkspace  VariableName=sig_exp_002_017  SaveFormat=Structure With Time
  ToWs_Req_Bus_Sig27 : ToWorkspace  VariableName=sig_exp_002_018  SaveFormat=Structure With Time
  ToWs_Req_Bus_Sig28 : ToWorkspace  VariableName=sig_exp_002_019  SaveFormat=Structure With Time
  ToWs_Req_Bus_Sig29 : ToWorkspace  VariableName=sig_exp_002_020  SaveFormat=Structure With Time
  ToWs_Req_Bus_Sig3 : ToWorkspace  VariableName=sig_req_002_003  SaveFormat=Structure With Time
  ToWs_Req_Bus_Sig30 : ToWorkspace  VariableName=sig_exp_002_021  SaveFormat=Structure With Time
  ToWs_Req_Bus_Sig31 : ToWorkspace  VariableName=sig_exp_002_022  SaveFormat=Structure With Time
  ToWs_Req_Bus_Sig32 : ToWorkspace  VariableName=sig_exp_002_023  SaveFormat=Structure With Time
  ToWs_Req_Bus_Sig33 : ToWorkspace  VariableName=sig_exp_002_024  SaveFormat=Structure With Time
  ToWs_Req_Bus_Sig34 : ToWorkspace  VariableName=sig_exp_002_025  SaveFormat=Structure With Time
  ToWs_Req_Bus_Sig35 : ToWorkspace  VariableName=sig_exp_002_026  SaveFormat=Structure With Time
  ToWs_Req_Bus_Sig36 : ToWorkspace  VariableName=sig_exp_002_027  SaveFormat=Structure With Time
  ToWs_Req_Bus_Sig37 : ToWorkspace  VariableName=sig_exp_002_028  SaveFormat=Structure With Time
  ToWs_Req_Bus_Sig4 : ToWorkspace  VariableName=sig_req_002_004  SaveFormat=Structure With Time
  ToWs_Req_Bus_Sig5 : ToWorkspace  VariableName=sig_req_002_005  SaveFormat=Structure With Time
  ToWs_Req_Bus_Sig6 : ToWorkspace  VariableName=sig_req_002_006  SaveFormat=Structure With Time
  ToWs_Req_Bus_Sig7 : ToWorkspace  VariableName=sig_req_002_007  SaveFormat=Structure With Time
  ToWs_Req_Bus_Sig8 : ToWorkspace  VariableName=sig_req_002_008  SaveFormat=Structure With Time
  ToWs_Req_Bus_Sig9 : ToWorkspace  VariableName=sig_req_002_009  SaveFormat=Structure With Time
  ToWs_Result_Bus_Sig1 : ToWorkspace  VariableName=sig_result_002_001  SaveFormat=Structure With Time
  ToWs_Result_Bus_Sig10 : ToWorkspace  VariableName=sig_result_002_010  SaveFormat=Structure With Time
  ToWs_Result_Bus_Sig11 : ToWorkspace  VariableName=sig_result_002_011  SaveFormat=Structure With Time
  ToWs_Result_Bus_Sig12 : ToWorkspace  VariableName=sig_result_002_012  SaveFormat=Structure With Time
  ToWs_Result_Bus_Sig13 : ToWorkspace  VariableName=sig_result_002_013  SaveFormat=Structure With Time
  ToWs_Result_Bus_Sig14 : ToWorkspace  VariableName=sig_result_002_014  SaveFormat=Structure With Time
  ToWs_Result_Bus_Sig15 : ToWorkspace  VariableName=sig_result_002_015  SaveFormat=Structure With Time
  ToWs_Result_Bus_Sig16 : ToWorkspace  VariableName=sig_result_002_016  SaveFormat=Structure With Time
  ToWs_Result_Bus_Sig17 : ToWorkspace  VariableName=sig_result_002_017  SaveFormat=Structure With Time
  ToWs_Result_Bus_Sig18 : ToWorkspace  VariableName=sig_result_002_018  SaveFormat=Structure With Time
  ToWs_Result_Bus_Sig19 : ToWorkspace  VariableName=sig_result_002_019  SaveFormat=Structure With Time
  ToWs_Result_Bus_Sig2 : ToWorkspace  VariableName=sig_result_002_002  SaveFormat=Structure With Time
  ToWs_Result_Bus_Sig20 : ToWorkspace  VariableName=sig_result_002_020  SaveFormat=Structure With Time
  ToWs_Result_Bus_Sig21 : ToWorkspace  VariableName=sig_result_002_021  SaveFormat=Structure With Time
  ToWs_Result_Bus_Sig22 : ToWorkspace  VariableName=sig_result_002_022  SaveFormat=Structure With Time
  ToWs_Result_Bus_Sig23 : ToWorkspace  VariableName=sig_result_002_023  SaveFormat=Structure With Time
  ToWs_Result_Bus_Sig24 : ToWorkspace  VariableName=sig_result_002_024  SaveFormat=Structure With Time
  ToWs_Result_Bus_Sig25 : ToWorkspace  VariableName=sig_result_002_025  SaveFormat=Structure With Time
  ToWs_Result_Bus_Sig26 : ToWorkspace  VariableName=sig_result_002_026  SaveFormat=Structure With Time
  ToWs_Result_Bus_Sig27 : ToWorkspace  VariableName=sig_result_002_027  SaveFormat=Structure With Time
  ToWs_Result_Bus_Sig28 : ToWorkspace  VariableName=sig_result_002_028  SaveFormat=Structure With Time
  ToWs_Result_Bus_Sig3 : ToWorkspace  VariableName=sig_result_002_003  SaveFormat=Structure With Time
  ToWs_Result_Bus_Sig4 : ToWorkspace  VariableName=sig_result_002_004  SaveFormat=Structure With Time
  ToWs_Result_Bus_Sig5 : ToWorkspace  VariableName=sig_result_002_005  SaveFormat=Structure With Time
  ToWs_Result_Bus_Sig6 : ToWorkspace  VariableName=sig_result_002_006  SaveFormat=Structure With Time
  ToWs_Result_Bus_Sig7 : ToWorkspace  VariableName=sig_result_002_007  SaveFormat=Structure With Time
  ToWs_Result_Bus_Sig8 : ToWorkspace  VariableName=sig_result_002_008  SaveFormat=Structure With Time
  ToWs_Result_Bus_Sig9 : ToWorkspace  VariableName=sig_result_002_009  SaveFormat=Structure With Time
  specifyOutputs : Subsystem
  result : Outport
  wires:
  sig_Req_Bus/1 -> BS/1, specifyOutputs/1(sig_Req_Bus)
  BS/1 -> ToWs_Req_Bus_Sig1/1  "<testSig_Epm_nEng>"
  BS/2 -> ToWs_Req_Bus_Sig2/1  "<testSig_PT_rGrip>"
  BS/3 -> ToWs_Req_Bus_Sig3/1  "<testSig_GlbDa_rTrqTot>"
  BS/4 -> ToWs_Req_Bus_Sig4/1  "<testSig_PthSet_trqInrSet>"
  BS/5 -> ToWs_Req_Bus_Sig5/1  "<testSig_PthLead_trqInrCurr>"
  BS/6 -> ToWs_Req_Bus_Sig6/1  "<testSig_PthLead_trqInrLead>"
  BS/7 -> ToWs_Req_Bus_Sig7/1  "<testSig_CEngDsT_t>"
  BS/8 -> ToWs_Req_Bus_Sig8/1  "<testSig_Oil_tSwmp>"
  BS/9 -> ToWs_Req_Bus_Sig9/1  "<testSig_EngDa_tEng>"
  BS/10 -> ToWs_Req_Bus_Sig10/1  "<testSig_HLSDem_facFdbkHi>"
  BS/11 -> ToWs_Req_Bus_Sig11/1  "<testSig_HLSDem_facFdbkLo>"
  BS/12 -> ToWs_Req_Bus_Sig12/1  "<testSig_HLSDem_facFdbkTrqLosLo>"
  BS/13 -> ToWs_Req_Bus_Sig13/1  "<testSig_HLSDem_facFdbkTrqLosHi>"
  BS/14 -> ToWs_Req_Bus_Sig14/1  "<testSig_HLSDem_tiFltTrqLosEstCurr>"
  BS/15 -> ToWs_Req_Bus_Sig15/1  "<testSig_HLSDem_InrtVehCurr>"
  BS/16 -> ToWs_Req_Bus_Sig16/1  "<testSig_HLSDem_dnAccLim>"
  BS/17 -> ToWs_Req_Bus_Sig17/1  "<testSig_HLSDem_dnDeclLim>"
  BS/18 -> ToWs_Req_Bus_Sig18/1  "<testSig_HLSDem_KpLoCurr_mp>"
  BS/19 -> ToWs_Req_Bus_Sig19/1  "<testSig_HLSDem_KpPosLoCurr_mp>"
  BS/20 -> ToWs_Req_Bus_Sig20/1  "<testSig_HLSDem_KpNegLoCurr_mp>"
  BS/21 -> ToWs_Req_Bus_Sig21/1  "<testSig_HLSDem_PWinPosLoCurr_mp>"
  BS/22 -> ToWs_Req_Bus_Sig22/1  "<testSig_HLSDem_PWinNegLoCurr_mp>"
  BS/23 -> ToWs_Req_Bus_Sig23/1  "<testSig_HLSDem_KiLoCurr_mp>"
  BS/24 -> ToWs_Req_Bus_Sig24/1  "<testSig_HLSDem_KiPosLoCurr_mp>"
  BS/25 -> ToWs_Req_Bus_Sig25/1  "<testSig_HLSDem_KiNegLoCurr_mp>"
  BS/26 -> ToWs_Req_Bus_Sig26/1  "<testSig_HLSDem_IWinPosLoCurr_mp>"
  BS/27 -> ToWs_Req_Bus_Sig27/1  "<testSig_HLSDem_IWinNegLoCurr_mp>"
  BS/28 -> ToWs_Req_Bus_Sig28/1  "<testSig_HLSDem_KpHiCurr_mp>"
  BS/29 -> ToWs_Req_Bus_Sig29/1  "<testSig_HLSDem_KpPosHiCurr_mp>"
  BS/30 -> ToWs_Req_Bus_Sig30/1  "<testSig_HLSDem_KpNegHiCurr_mp>"
  BS/31 -> ToWs_Req_Bus_Sig31/1  "<testSig_HLSDem_PWinPosHiCurr_mp>"
  BS/32 -> ToWs_Req_Bus_Sig32/1  "<testSig_HLSDem_PWinNegHiCurr_mp>"
  BS/33 -> ToWs_Req_Bus_Sig33/1  "<testSig_HLSDem_KiHiCurr_mp>"
  BS/34 -> ToWs_Req_Bus_Sig34/1  "<testSig_HLSDem_KiPosHiCurr_mp>"
  BS/35 -> ToWs_Req_Bus_Sig35/1  "<testSig_HLSDem_KiNegHiCurr_mp>"
  BS/36 -> ToWs_Req_Bus_Sig36/1  "<testSig_HLSDem_IWinPosHiCurr_mp>"
  BS/37 -> ToWs_Req_Bus_Sig37/1  "<testSig_HLSDem_IWinNegHiCurr_mp>"
  sig_Result_Bus/1 -> BS_Result/1, specifyOutputs/2(sig_Result_Bus)
  BS_Result/1 -> ToWs_Result_Bus_Sig1/1  "<HLSDem_facFdbkHi>"
  BS_Result/2 -> ToWs_Result_Bus_Sig2/1  "<HLSDem_facFdbkLo>"
  BS_Result/3 -> ToWs_Result_Bus_Sig3/1  "<HLSDem_facFdbkTrqLosLo>"
  BS_Result/4 -> ToWs_Result_Bus_Sig4/1  "<HLSDem_facFdbkTrqLosHi>"
  BS_Result/5 -> ToWs_Result_Bus_Sig5/1  "<HLSDem_tiFltTrqLosEstCurr>"
  BS_Result/6 -> ToWs_Result_Bus_Sig6/1  "<HLSDem_InrtVehCurr>"
  BS_Result/7 -> ToWs_Result_Bus_Sig7/1  "<HLSDem_dnAccLim>"
  BS_Result/8 -> ToWs_Result_Bus_Sig8/1  "<HLSDem_dnDeclLim>"
  BS_Result/9 -> ToWs_Result_Bus_Sig9/1  "<HLSDem_KpLoCurr_mp>"
  BS_Result/10 -> ToWs_Result_Bus_Sig10/1  "<HLSDem_KpPosLoCurr_mp>"
  BS_Result/11 -> ToWs_Result_Bus_Sig11/1  "<HLSDem_KpNegLoCurr_mp>"
  BS_Result/12 -> ToWs_Result_Bus_Sig12/1  "<HLSDem_PWinPosLoCurr_mp>"
  BS_Result/13 -> ToWs_Result_Bus_Sig13/1  "<HLSDem_PWinNegLoCurr_mp>"
  BS_Result/14 -> ToWs_Result_Bus_Sig14/1  "<HLSDem_KiLoCurr_mp>"
  BS_Result/15 -> ToWs_Result_Bus_Sig15/1  "<HLSDem_KiPosLoCurr_mp>"
  BS_Result/16 -> ToWs_Result_Bus_Sig16/1  "<HLSDem_KiNegLoCurr_mp>"
  BS_Result/17 -> ToWs_Result_Bus_Sig17/1  "<HLSDem_IWinPosLoCurr_mp>"
  BS_Result/18 -> ToWs_Result_Bus_Sig18/1  "<HLSDem_IWinNegLoCurr_mp>"
  BS_Result/19 -> ToWs_Result_Bus_Sig19/1  "<HLSDem_KpHiCurr_mp>"
  BS_Result/20 -> ToWs_Result_Bus_Sig20/1  "<HLSDem_KpPosHiCurr_mp>"
  BS_Result/21 -> ToWs_Result_Bus_Sig21/1  "<HLSDem_KpNegHiCurr_mp>"
  BS_Result/22 -> ToWs_Result_Bus_Sig22/1  "<HLSDem_PWinPosHiCurr_mp>"
  BS_Result/23 -> ToWs_Result_Bus_Sig23/1  "<HLSDem_PWinNegHiCurr_mp>"
  BS_Result/24 -> ToWs_Result_Bus_Sig24/1  "<HLSDem_KiHiCurr_mp>"
  BS_Result/25 -> ToWs_Result_Bus_Sig25/1  "<HLSDem_KiPosHiCurr_mp>"
  BS_Result/26 -> ToWs_Result_Bus_Sig26/1  "<HLSDem_KiNegHiCurr_mp>"
  BS_Result/27 -> ToWs_Result_Bus_Sig27/1  "<HLSDem_IWinPosHiCurr_mp>"
  BS_Result/28 -> ToWs_Result_Bus_Sig28/1  "<HLSDem_IWinNegHiCurr_mp>"
  specifyOutputs/1(result) -> result/1
